simulink model "random_integer_input"  (R2024a)
settings: Solver=VariableStepAuto  StartTime=0.0  StopTime=inf  RelTol=1e-3
libraries: commrflib2 x2, commchan3 x1, commdigbbndpm3 x1, commfilt2 x1, commrandsrc3 x1, dspnetwork x1
settings Model: Creator=digital  LastModifiedBy=digital

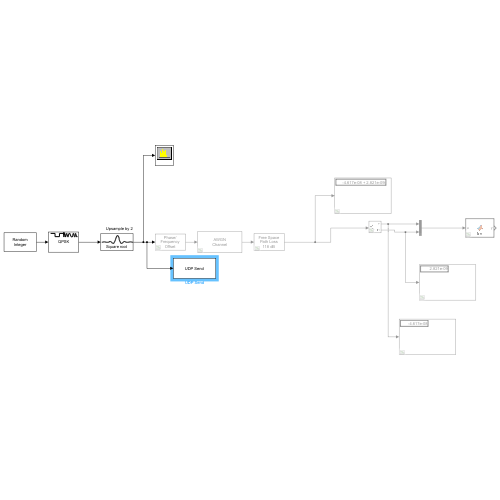
[thumbnail: Simulink's stored preview of the top-level diagram]
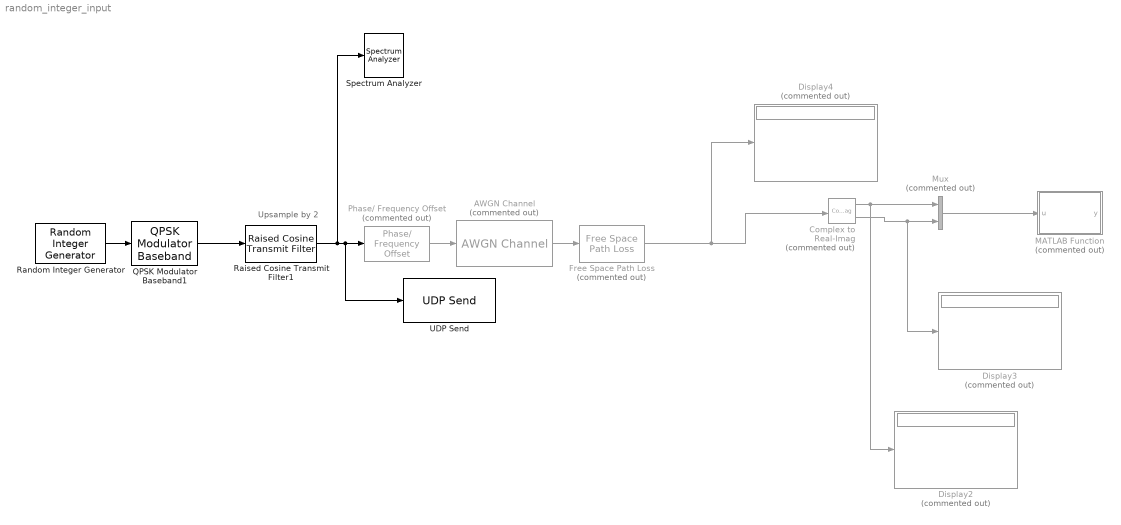
== system random_integer_input ==
  note: Upsample by 2
  AWGN Channel : commchan3/AWGN Channel  Commented=on  LegacyMode=off  NoiseMethod="Signal to noise ratio  (SNR)"  noiseMode="Signal to noise ratio  (SNR)"  EbNo=10  EsNo=10  SNR=30  BitsPerSymbol=1  SignalPower=1  SamplesPerSymbol=1  SymbolPeriod=1  VarianceSource=Parameter  Variance=1  RandomStream=Global stream  Seed=67  SimulateUsing=Interpreted execution
  Complex to Real-Imag : ComplexToRealImag  Commented=on
  Display2 : Display  Commented=on
  Display3 : Display  Commented=on
  Display4 : Display  Commented=on
  Free Space Path Loss : commrflib2/Free Space Path Loss  Commented=on  mode=Distance and Frequency  dB=10  d=10  fc=1920
  MATLAB Function : MATLAB Function  Commented=on  TreatAsAtomicUnit=on
  Mux : Mux  Commented=on  Inputs=2
  Phase/ Frequency Offset : commrflib2/Phase// Frequency Offset  Commented=on  phaseOffset=0  freqPort=off  freqOffset=0
  QPSK Modulator Baseband1 : commdigbbndpm3/QPSK Modulator Baseband  InType=Integer  Enc=Gray  Ph=pi/4  outDtype=double  outWordLen=16  outUDDataType=sfix(16)  outFracLenMode=Best precision  outFracLen=15  outDataTypeStr=double  outLastDataTypeStr=double
  Raised Cosine Transmit Filter1 : commfilt2/Raised Cosine Transmit Filter  filtType=Square root  R=0.2  filtSpan=10  N=10  filterGain=1  RateOptions=Allow multirate processing  framing=Mute  checkCoeff=off  variableName=rcTxFilt1  checkGain=Normalized  sampMode=Mute  saveAsFlag=0  currentFiltSpan=10  D=(10)/2  launchFVT=on  roundingMode=Floor  overflowMode=off  coeffDataTypeStr=Inherit: Same word length as input  coeffMin=[]  coeffMax=[]  coeffLastDataTypeStr=Inherit: Same word length as input  outputDataTypeStr=Inherit: Same as accumulator  outputMin=[]  outputMax=[]  outputLastDataTypeStr=Inherit: Same as accumulator
  Random Integer Generator : commrandsrc3/Random Integer Generator  SetSize=4  SeedSource=Auto  Seed=0  SampleTime=1/1e3  SamplesPerFrame=1  OutputDataType=double  SimulateUsing=Interpreted execution
  Spectrum Analyzer : SpectrumAnalyzer  WindowPosition=[1.000000,49.000000,2048.000000,1080.000000,]  ScopeFrameLocation=window  Span=2000000  YLimits=[-89.35883318,11.30544811]  SelectedToolstripTab=spectrumAnalyzerToolstrip.spectrumTab
  UDP Send : dspnetwork/UDP Send  remoteURL='192.168.1.1'  remotePort=8001  localURL='0.0.0.0'  localPortSource=Automatically determine  localPort=-1  sendBufferSize=8192  sampletime=-1  blockPlatform=[]  separateLengthPort=0
      settings: LibrarySourceBlock=dspsnks4/UDP Send
  wires:
  Mux/1 -> MATLAB Function/1(u)
  QPSK Modulator Baseband1/1 -> Raised Cosine Transmit Filter1/1
  Raised Cosine Transmit Filter1/1 -> Spectrum Analyzer/1, UDP Send/1, Phase/ Frequency Offset/1
  AWGN Channel/1 -> Free Space Path Loss/1
  Phase/ Frequency Offset/1 -> AWGN Channel/1
  Free Space Path Loss/1 -> Display4/1, Complex to Real-Imag/1
  Complex to Real-Imag/2 -> Display3/1, Mux/2
  Complex to Real-Imag/1 -> Mux/1, Display2/1
  Random Integer Generator/1 -> QPSK Modulator Baseband1/1

== matlab function random_integer_input/MATLAB Function ==
  data: u input; y output
function y = fcn(u)

y = typecast(u,"uint8");
